simulink model "NoVCU"  (R2024b)
settings: configuration reference "VehicleFixed10ms" (kept outside this file)
undefined symbols (not defined in the file): PlntEngTqMax
settings Model: DataDictionary=VirtualVehicleTemplate.sldd  ModifiedByFormat=The MathWorks, Inc.  Creator=The MathWorks, Inc.  LastModifiedBy=The MathWorks, Inc.
settings ConfigSetRef: SourceName=VehicleFixed10ms

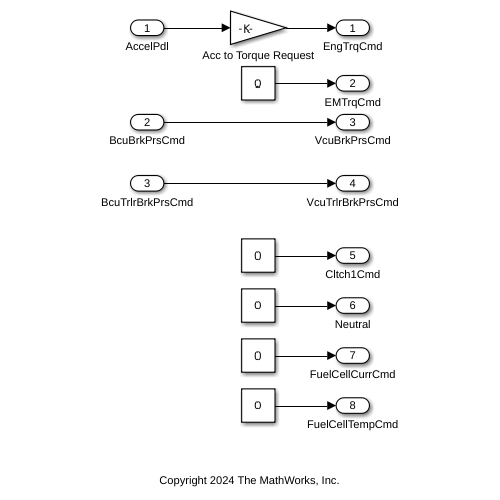
[thumbnail: Simulink's stored preview of the top-level diagram]
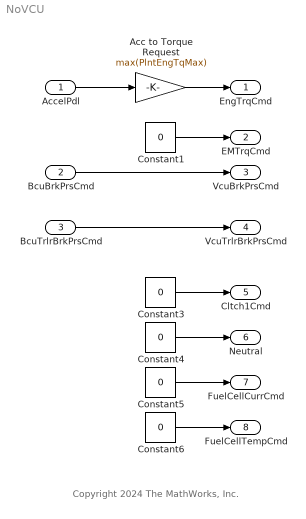
== system NoVCU ==
  note: Copyright 2024 The MathWorks, Inc.
  AccelPdl : Inport
  BcuBrkPrsCmd : Inport  Port=2  SampleTime=0.01
  BcuTrlrBrkPrsCmd : Inport  Port=3  SampleTime=0.01
  Acc to Torque Request : Gain  Gain=max(PlntEngTqMax)
  Constant{1,3..6} (5 alike) : Constant  Value=0  SampleTime=-1
  EngTrqCmd : Outport  OutDataTypeStr=double  PortDimensions=1  SampleTime=[0.01,0]  VectorParamsAs1DForOutWhenUnconnected=off
  EMTrqCmd : Outport  Port=2  VectorParamsAs1DForOutWhenUnconnected=off
  VcuBrkPrsCmd : Outport  Port=3  PortDimensions=4  VectorParamsAs1DForOutWhenUnconnected=off
  VcuTrlrBrkPrsCmd : Outport  Port=4  PortDimensions=6  VectorParamsAs1DForOutWhenUnconnected=off
  Cltch1Cmd : Outport  Port=5  PortDimensions=1  SampleTime=[0.01,0]  VectorParamsAs1DForOutWhenUnconnected=off
  Neutral : Outport  Port=6  PortDimensions=1  SampleTime=[0.01,0]  VectorParamsAs1DForOutWhenUnconnected=off
  FuelCellCurrCmd : Outport  Port=7  SampleTime=.01
  FuelCellTempCmd : Outport  Port=8
  wires:
  BcuTrlrBrkPrsCmd/1 -> VcuTrlrBrkPrsCmd/1
  Constant1/1 -> EMTrqCmd/1
  Constant3/1 -> Cltch1Cmd/1
  AccelPdl/1 -> Acc to Torque Request/1
  Constant5/1 -> FuelCellCurrCmd/1
  Acc to Torque Request/1 -> EngTrqCmd/1
  BcuBrkPrsCmd/1 -> VcuBrkPrsCmd/1
  Constant4/1 -> Neutral/1
  Constant6/1 -> FuelCellTempCmd/1
